simulink model "Playground"  (R2013a)
settings: Solver=ode45  StartTime=0.0  StopTime=10/1200  RelTol=1e-3
libraries: dsparch4 x2, commrandsrc2 x1, commsynccomp2 x1
settings Model: Creator=Cedric  LastModifiedBy=Cedric

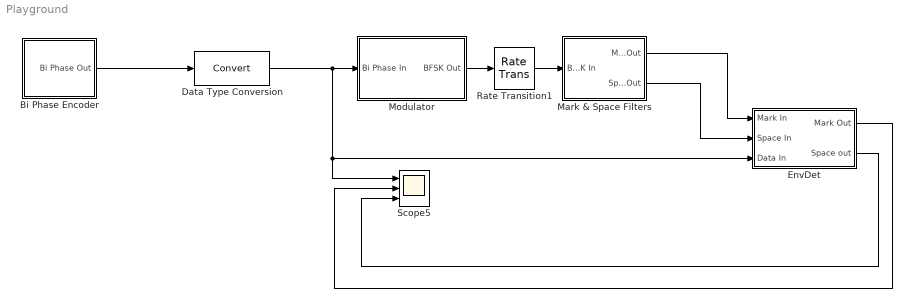
== system Playground ==
  Bi Phase Encoder : Subsystem
  Data Type Conversion : DataTypeConversion
  EnvDet : Subsystem
  Mark & Space Filters : Subsystem
  Modulator : Subsystem
  Rate Transition1 : RateTransition  OutPortSampleTime=1/(1200*256)
  Scope5 : Scope  NumInputPorts=3
      settings: YMin=-0.5~-5~-5  YMax=1.5~5~5
  wires:
  Bi Phase Encoder/1(Bi Phase Out) -> Data Type Conversion/1
  Modulator/1(BFSK Out) -> Rate Transition1/1
  Data Type Conversion/1 -> Modulator/1(Bi Phase In), Scope5/1, EnvDet/3(Data In)
  Rate Transition1/1 -> Mark & Space Filters/1(BPFSK In)
  EnvDet/2(Space out) -> Scope5/3
  EnvDet/1(Mark Out) -> Scope5/2
  Mark & Space Filters/1(Mark Out) -> EnvDet/1(Mark In)
  Mark & Space Filters/2(Space Out) -> EnvDet/2(Space In)

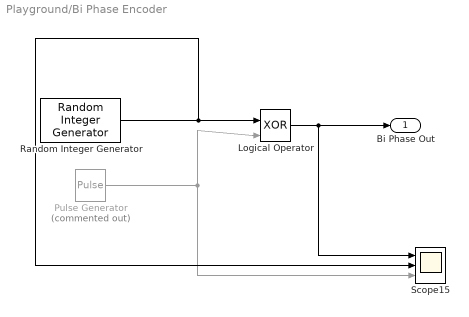
== system Playground/Bi Phase Encoder ==
  Logical Operator : Logic  Operator=XOR  IconShape=distinctive  AllPortsSameDT=off  OutDataTypeStr=boolean
  Pulse Generator : DiscretePulseGenerator  Commented=on  Period=256  PulseWidth=128  SampleTime=1/(1200*256)
  Random Integer Generator : commrandsrc2/Random Integer Generator  mul=1  seed=randseed  Ts=1/1200  frameBased=off  sampPerFrame=1  orient=off  outDataType=double
  Scope15 : Scope  NumInputPorts=3
      settings: TimeRange=0.005  YMin=-5~-5~-5  YMax=5~5~5  SaveName=FSK4
  Bi Phase Out : Outport
  wires:
  Pulse Generator/1 -> Logical Operator/2, Scope15/3
  Random Integer Generator/1 -> Scope15/2, Logical Operator/1
  Logical Operator/1 -> Scope15/1, Bi Phase Out/1

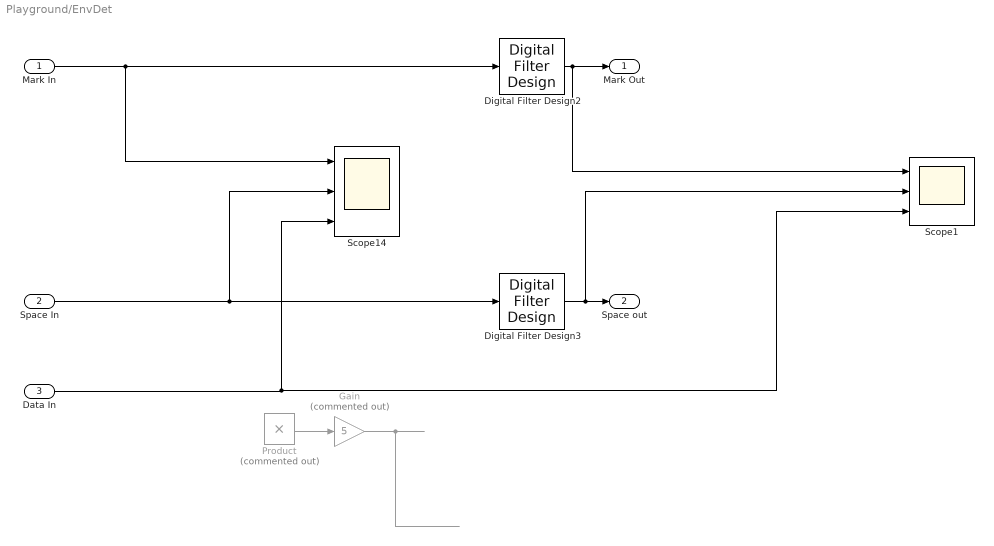
== system Playground/EnvDet ==
  Mark In : Inport
  Space In : Inport  Port=2
  Data In : Inport  Port=3
  Digital Filter Design2 : dsparch4/Digital Filter Design  mwdsp_browser_bugfix_var=off
  Digital Filter Design3 : dsparch4/Digital Filter Design  mwdsp_browser_bugfix_var=off
  Gain : Gain  Commented=on  Gain=5
  Product : Product  Commented=on
  Scope1 : Scope  NumInputPorts=3
      settings: YMin=-0.1~-0.1~-5  YMax=0.1~0.1~5
  Scope14 : Scope  NumInputPorts=3
      settings: YMin=-0.1~-0.1~-5  YMax=0.1~0.1~5  SaveName=ScopeData9
  Mark Out : Outport
  Space out : Outport  Port=2
  wires:
  Data In/1 -> Scope1/3, Scope14/3
  Mark In/1 -> Digital Filter Design2/1, Scope14/1
  Space In/1 -> Digital Filter Design3/1, Scope14/2
  Product/1 -> Gain/1
  Gain/1 -> ?
  Digital Filter Design2/1 -> Scope1/1, Mark Out/1
  Digital Filter Design3/1 -> Scope1/2, Space out/1

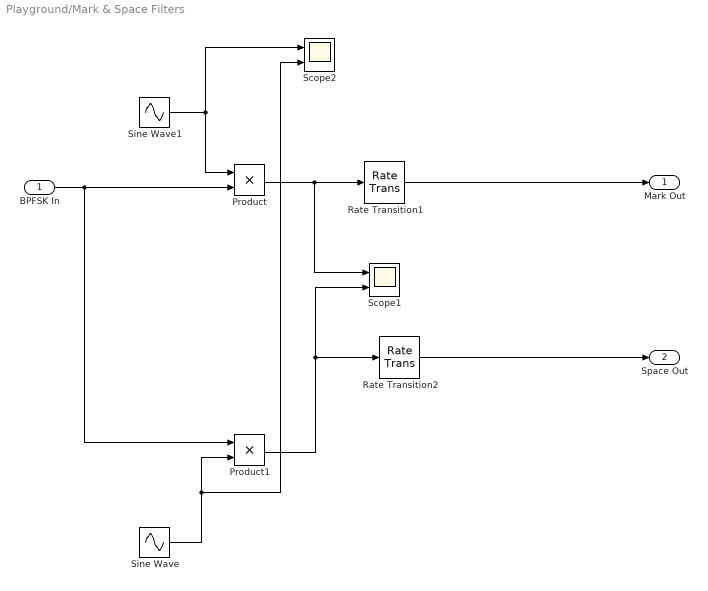
== system Playground/Mark & Space Filters ==
  BPFSK In : Inport
  Product : Product
  Product1 : Product
  Rate Transition1 : RateTransition  OutPortSampleTime=1/(1200*256)
  Rate Transition2 : RateTransition  OutPortSampleTime=1/(1200*256)
  Scope1 : Scope  NumInputPorts=2
      settings: YMin=-5~-5  YMax=5~5  SaveName=ScopeData2
  Scope2 : Scope  NumInputPorts=2
      settings: YMin=-5~-5  YMax=5~5  SaveName=ScopeData3
  Sine Wave : Sin  SineType=Sample based  Samples=256  SampleTime=1/(1200*426.667)  Offset=128
  Sine Wave1 : Sin  SineType=Sample based  Samples=256  SampleTime=1/(1200*256)  Offset=128
  Mark Out : Outport
  Space Out : Outport  Port=2
  wires:
  BPFSK In/1 -> Product1/1, Product/2
  Product/1 -> Rate Transition1/1, Scope1/1
  Sine Wave1/1 -> Scope2/1, Product/1
  Product1/1 -> Scope1/2, Rate Transition2/1
  Sine Wave/1 -> Product1/2, Scope2/2
  Rate Transition1/1 -> Mark Out/1
  Rate Transition2/1 -> Space Out/1

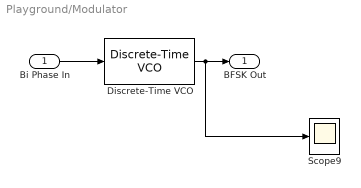
== system Playground/Modulator ==
  Bi Phase In : Inport
  Discrete-Time VCO : commsynccomp2/Discrete-Time VCO  Ac=5  Fc=1200  Kc=1000  Ph=0  ts=1/(1200*256)
  Scope9 : Scope
      settings: TimeRange=0.005  SaveName=FSK1
  BFSK Out : Outport
  wires:
  Bi Phase In/1 -> Discrete-Time VCO/1
  Discrete-Time VCO/1 -> Scope9/1, BFSK Out/1
